simulink model "RFSnoPFC"  (R2024a)
settings: Solver=VariableStepAuto  StartTime=0.0  StopTime=0.1  MaxStep=1e-6  RelTol=1e-3
undefined symbols (not defined in the file or in its folder): b, c
libraries: cstblocks x4
settings Model: Creator=FactCore  LastModifiedBy=FactCore

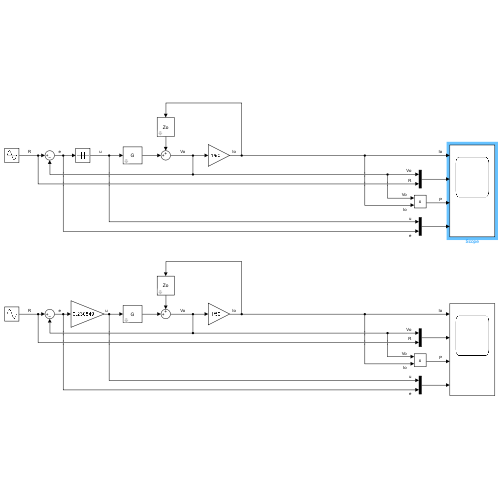
[thumbnail: Simulink's stored preview of the top-level diagram]
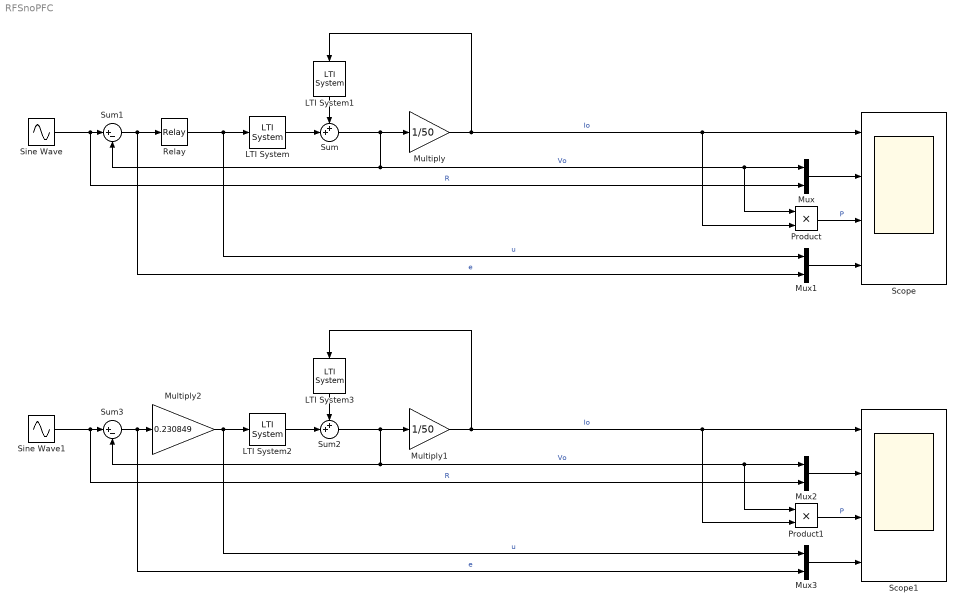
== system RFSnoPFC ==
  LTI System : cstblocks/LTI System  sys=G  IC=[]  PadeOrder=0
  LTI System1 : cstblocks/LTI System  sys=Zo  IC=[]  PadeOrder=0
  LTI System2 : cstblocks/LTI System  sys=G  IC=[]  PadeOrder=0
  LTI System3 : cstblocks/LTI System  sys=Zo  IC=[]  PadeOrder=0
  Multiply : Gain  Gain=1/50
  Multiply1 : Gain  Gain=1/50
  Multiply2 : Gain  Gain=0.230849
  Mux{,1..3} (4 alike) : Mux  Inputs=2
  Product : Product
  Product1 : Product
  Relay : Relay  OnSwitchValue=b  OffSwitchValue=-b  OffOutputValue=-c
  Scope : Scope  NumInputPorts=4
  Scope1 : Scope  NumInputPorts=4
  Sine Wave : Sin  Amplitude=230*sqrt(2)  Frequency=2*pi*50  SampleTime=0
  Sine Wave1 : Sin  Amplitude=230*sqrt(2)  Frequency=2*pi*50  SampleTime=0
  Sum : Sum  Inputs=++|
  Sum1 : Sum  Inputs=|+-
  Sum2 : Sum  Inputs=++|
  Sum3 : Sum  Inputs=|+-
  wires:
  LTI System/1 -> Sum/2
  LTI System1/1 -> Sum/1
  Sum/1 -> Multiply/1, Sum1/2, Product/1, Mux/1  "Vo"
  Multiply/1 -> Product/2, Scope/1, LTI System1/1  "Io"
  Relay/1 -> Mux1/1, LTI System/1  "u"
  Product/1 -> Scope/3  "P"
  Sum1/1 -> Mux1/2, Relay/1  "e"
  Sine Wave/1 -> Mux/2, Sum1/1  "R"
  Mux/1 -> Scope/2
  Mux1/1 -> Scope/4
  Mux3/1 -> Scope1/4
  Mux2/1 -> Scope1/2
  Sine Wave1/1 -> Sum3/1, Mux2/2  "R"
  Sum3/1 -> Multiply2/1, Mux3/2  "e"
  Product1/1 -> Scope1/3  "P"
  Multiply2/1 -> LTI System2/1, Mux3/1  "u"
  Multiply1/1 -> LTI System3/1, Scope1/1, Product1/2  "Io"
  Sum2/1 -> Mux2/1, Product1/1, Sum3/2, Multiply1/1  "Vo"
  LTI System3/1 -> Sum2/1
  LTI System2/1 -> Sum2/2
